simulink model "Simulation_ipmsm_velocity_control"  (R2023a)
settings: Solver=FixedStepDiscrete  StartTime=0.0  StopTime=2  FixedStep=Ts  RelTol=1e-3  EnableMultiTasking=on
PreLoadFcn:
  | ee_ipmsm_velocity_control_data;
StopFcn:
  | ee_addSimlogTimeStamp(bdroot)
undefined symbols (not defined in the file): Ld, Lq, p, psim, Ts, VDC_VECT, Vnom
libraries: nesl_utility x14, fl_lib x11, mcbcontrolslib x9, ee_lib x4, simulink x2, batteryecm_lib x1, eePmsmCurrentController x1, eeTransforms x1, eePmsmCurrentReferenceGen x1, eeVelocityController x1, eePwmGeneratorTwoLevel x1, SignalEditorBlockLib x1
(part 2 of 2)

== system Simulation_ipmsm_velocity_control/Control/Current Control/Subsystem1/Subsystem2/HPF_Calc ==
  In1 : Inport
  VfHpf_FilterCornerFreq_Hz : Inport  Port=2
  VfHpf_FilterTs_s : Inport  Port=3
  HPF_Coef_Calc : Subsystem
  HPF_Module : Subsystem
  HPF : Outport
  wires:
  VfHpf_FilterCornerFreq_Hz/1 -> HPF_Coef_Calc/1(VfHpf_FilterCornerFreq_Hz)
  HPF_Coef_Calc/2(VfHpf_FilterD_coef) -> HPF_Module/3(VfHpf_FilterD_coef)
  HPF_Coef_Calc/1(VfHpf_FilterN_coef) -> HPF_Module/2(VfHpf_FilterN_coef)
  HPF_Module/1(HPF) -> HPF/1
  In1/1 -> HPF_Module/1(In1)
  VfHpf_FilterTs_s/1 -> HPF_Coef_Calc/2(VfHpf_FilterTs_s)

== system Simulation_ipmsm_velocity_control/Control/Current Control/Subsystem1/Subsystem3/HPF_Calc ==
  In1 : Inport
  VfHpf_FilterCornerFreq_Hz : Inport  Port=2
  VfHpf_FilterTs_s : Inport  Port=3
  HPF_Coef_Calc : Subsystem
  HPF_Module : Subsystem
  HPF : Outport
  wires:
  VfHpf_FilterCornerFreq_Hz/1 -> HPF_Coef_Calc/1(VfHpf_FilterCornerFreq_Hz)
  HPF_Coef_Calc/2(VfHpf_FilterD_coef) -> HPF_Module/3(VfHpf_FilterD_coef)
  HPF_Coef_Calc/1(VfHpf_FilterN_coef) -> HPF_Module/2(VfHpf_FilterN_coef)
  HPF_Module/1(HPF) -> HPF/1
  In1/1 -> HPF_Module/1(In1)
  VfHpf_FilterTs_s/1 -> HPF_Coef_Calc/2(VfHpf_FilterTs_s)

== system Simulation_ipmsm_velocity_control/Control/Current Control/SVM_PU/T1_T2_Calc/Subsystem1/Enabled Subsystem ==
  Z : Inport
  Y : Inport  Port=2
  Action Port : ActionPort  ActionPortLabel=case [ 1 ]:
  T4 : Outport
  T6 : Outport  Port=2
  wires:
  Z/1 -> T4/1
  Y/1 -> T6/1

== system Simulation_ipmsm_velocity_control/Control/Current Control/SVM_PU/T1_T2_Calc/Subsystem1/Enabled Subsystem1 ==
  Y : Inport
  X : Inport  Port=2
  Action Port : ActionPort  ActionPortLabel=case [ 2 ]:
  Gain : Gain  Gain=-1
  T4 : Outport
  T6 : Outport  Port=2
  wires:
  Y/1 -> T4/1
  Gain/1 -> T6/1
  X/1 -> Gain/1

== system Simulation_ipmsm_velocity_control/Control/Current Control/SVM_PU/T1_T2_Calc/Subsystem1/Enabled Subsystem2 ==
  Z : Inport
  X : Inport  Port=2
  Action Port : ActionPort  ActionPortLabel=case [ 3 ]:
  Gain : Gain  Gain=-1
  T4 : Outport
  T6 : Outport  Port=2
  wires:
  Z/1 -> Gain/1
  X/1 -> T6/1
  Gain/1 -> T4/1

== system Simulation_ipmsm_velocity_control/Control/Current Control/SVM_PU/T1_T2_Calc/Subsystem1/Enabled Subsystem3 ==
  X : Inport
  Z : Inport  Port=2
  Action Port : ActionPort  ActionPortLabel=case [ 4 ]:
  Gain : Gain  Gain=-1
  T4 : Outport
  T6 : Outport  Port=2
  wires:
  X/1 -> Gain/1
  Z/1 -> T6/1
  Gain/1 -> T4/1

== system Simulation_ipmsm_velocity_control/Control/Current Control/SVM_PU/T1_T2_Calc/Subsystem1/Enabled Subsystem4 ==
  X : Inport
  Y : Inport  Port=2
  Action Port : ActionPort  ActionPortLabel=case [ 5 ]:
  Gain : Gain  Gain=-1
  T4 : Outport
  T6 : Outport  Port=2
  wires:
  Y/1 -> Gain/1
  X/1 -> T4/1
  Gain/1 -> T6/1

== system Simulation_ipmsm_velocity_control/Control/Current Control/SVM_PU/T1_T2_Calc/Subsystem1/Enabled Subsystem5 ==
  Y : Inport
  Z : Inport  Port=2
  Action Port : ActionPort  ActionPortLabel=case [ 6 ]:
  Gain : Gain  Gain=-1
  Gain1 : Gain  Gain=-1
  T4 : Outport
  T6 : Outport  Port=2
  wires:
  Y/1 -> Gain/1
  Z/1 -> Gain1/1
  Gain/1 -> T4/1
  Gain1/1 -> T6/1

== system Simulation_ipmsm_velocity_control/Control/Current Control/SVM_PU/T1_T2_Calc/Subsystem1/Enabled Subsystem6 ==
  Y : Inport
  Z : Inport  Port=2
  Action Port : ActionPort  ActionPortLabel=default:
  Gain : Gain  Gain=-1
  Gain1 : Gain  Gain=-1
  T4 : Outport
  T6 : Outport  Port=2
  wires:
  Y/1 -> Gain/1
  Z/1 -> Gain1/1
  Gain/1 -> T4/1
  Gain1/1 -> T6/1

== system Simulation_ipmsm_velocity_control/Control/Current Control/SVM_PU/T1_T2_Calc/Subsystem2/If Action Subsystem ==
  Bus_T4T6 : Inport
  Action Port : ActionPort  ActionPortLabel=else
  Bus Selector : BusSelector  OutputSignals=T4,T6
  Signal Copy1 : SignalConversion  OverrideOpt=off
  Signal Copy2 : SignalConversion  OverrideOpt=off
  T1 : Outport
  T2 : Outport  Port=2
  wires:
  Bus_T4T6/1 -> Bus Selector/1
  Bus Selector/1 -> Signal Copy1/1  "<T4>"
  Bus Selector/2 -> Signal Copy2/1  "<T6>"
  Signal Copy1/1 -> T1/1
  Signal Copy2/1 -> T2/1

== system Simulation_ipmsm_velocity_control/Control/Current Control/SVM_PU/T1_T2_Calc/Subsystem2/If Action Subsystem1 ==
  Bus_T4T6 : Inport
  Action Port : ActionPort  ActionPortLabel=elseif(u1 > 1)
  Add : Sum
  Bus Selector : BusSelector  OutputSignals=T4,T6
  Divide : Product  Inputs=*/
  Divide1 : Product  Inputs=/*
  T1 : Outport
  T2 : Outport  Port=2
  wires:
  Bus_T4T6/1 -> Bus Selector/1
  Bus Selector/1 -> Divide/1, Add/1  "<T4>"
  Bus Selector/2 -> Divide1/2, Add/2  "<T6>"
  Add/1 -> Divide1/1, Divide/2
  Divide/1 -> T1/1  "T1"
  Divide1/1 -> T2/1  "T2"

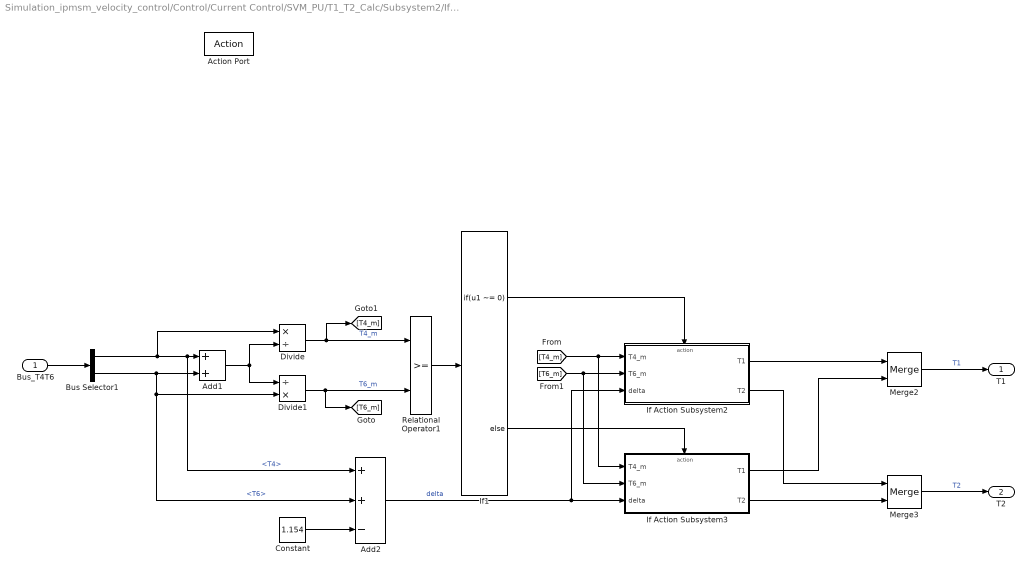
== system Simulation_ipmsm_velocity_control/Control/Current Control/SVM_PU/T1_T2_Calc/Subsystem2/If Action Subsystem2 ==
  Bus_T4T6 : Inport
  Action Port : ActionPort  ActionPortLabel=if(u1 > 1.154 )
  Add1 : Sum
  Add2 : Sum  Inputs=++-
  Bus Selector1 : BusSelector  OutputSignals=T4,T6
  Constant : Constant  Value=1.154  OutDataTypeStr=single
  Divide : Product  Inputs=*/
  Divide1 : Product  Inputs=/*
  If Action Subsystem2 : Subsystem  TreatAsAtomicUnit=on
  If Action Subsystem3 : Subsystem  TreatAsAtomicUnit=on
  If1 : If  IfExpression=u1 ~= 0
  Merge2 : Merge
  Merge3 : Merge
  Relational Operator1 : RelationalOperator  OutDataTypeStr=boolean  RndMeth=Simplest  InputSameDT=off
  T1 : Outport
  T2 : Outport  Port=2
  wires:
  Bus_T4T6/1 -> Bus Selector1/1
  Bus Selector1/2 -> Divide1/2, Add2/2, Add1/2  "<T6>"
  Divide/1 -> [T4_m], Relational Operator1/1  "T4_m"
  Bus Selector1/1 -> Divide/1, Add2/1, Add1/1  "<T4>"
  Divide1/1 -> [T6_m], Relational Operator1/2  "T6_m"
  Add1/1 -> Divide1/1, Divide/2
  Relational Operator1/1 -> If1/1
  Constant/1 -> Add2/3
  Add2/1 -> If Action Subsystem2/3(delta), If Action Subsystem3/3(delta)  "delta"
  If1/1 -> If Action Subsystem2/Action
  If1/2 -> If Action Subsystem3/Action
  If Action Subsystem2/1(T1) -> Merge2/1
  If Action Subsystem3/1(T1) -> Merge2/2
  If Action Subsystem3/2(T2) -> Merge3/2
  If Action Subsystem2/2(T2) -> Merge3/1
  Merge2/1 -> T1/1  "T1"
  Merge3/1 -> T2/1  "T2"
  [T4_m] -> If Action Subsystem3/1(T4_m), If Action Subsystem2/1(T4_m)
  [T6_m] -> If Action Subsystem3/2(T6_m), If Action Subsystem2/2(T6_m)

== system Simulation_ipmsm_velocity_control/Control/Current Control/Subsystem1/Subsystem2/HPF_Calc/HPF_Coef_Calc ==
  VfHpf_FilterCornerFreq_Hz : Inport
  VfHpf_FilterTs_s : Inport  Port=2
  Add : Sum
  Add1 : Sum  Inputs=+-
  Constant : Constant  Value=2*pi  OutDataTypeStr=single
  Constant1 : Constant  Value=2  OutDataTypeStr=single
  Divide : Product  Inputs=*/
  Divide1 : Product  Inputs=/*
  Product : Product  Inputs=3
  VfHpf_FilterN_coef : Outport
  VfHpf_FilterD_coef : Outport  Port=2
  wires:
  VfHpf_FilterCornerFreq_Hz/1 -> Product/1
  VfHpf_FilterTs_s/1 -> Product/2
  Constant/1 -> Product/3
  Product/1 -> Add1/2, Add/2  "Omiga0PrTs"
  Constant1/1 -> Add1/1, Divide/1, Add/1
  Add/1 -> Divide1/1, Divide/2
  Divide/1 -> VfHpf_FilterN_coef/1
  Add1/1 -> Divide1/2
  Divide1/1 -> VfHpf_FilterD_coef/1

== system Simulation_ipmsm_velocity_control/Control/Current Control/Subsystem1/Subsystem2/HPF_Calc/HPF_Module ==
  In1 : Inport
  VfHpf_FilterN_coef : Inport  Port=2
  VfHpf_FilterD_coef : Inport  Port=3
  Add : Sum  Inputs=+-
  Add1 : Sum
  Delay : Delay  DelayLength=1
  Delay1 : Delay  DelayLength=1
  Product : Product
  Product1 : Product
  HPF : Outport
  wires:
  In1/1 -> Delay/1, Add/1
  Delay/1 -> Add/2
  Add/1 -> Product/1
  VfHpf_FilterN_coef/1 -> Product/2
  Product/1 -> Add1/1
  Add1/1 -> Delay1/1, HPF/1
  VfHpf_FilterD_coef/1 -> Product1/1
  Product1/1 -> Add1/2
  Delay1/1 -> Product1/2

== system Simulation_ipmsm_velocity_control/Control/Current Control/Subsystem1/Subsystem3/HPF_Calc/HPF_Coef_Calc ==
  VfHpf_FilterCornerFreq_Hz : Inport
  VfHpf_FilterTs_s : Inport  Port=2
  Add : Sum
  Add1 : Sum  Inputs=+-
  Constant : Constant  Value=2*pi  OutDataTypeStr=single
  Constant1 : Constant  Value=2  OutDataTypeStr=single
  Divide : Product  Inputs=*/
  Divide1 : Product  Inputs=/*
  Product : Product  Inputs=3
  VfHpf_FilterN_coef : Outport
  VfHpf_FilterD_coef : Outport  Port=2
  wires:
  VfHpf_FilterCornerFreq_Hz/1 -> Product/1
  VfHpf_FilterTs_s/1 -> Product/2
  Constant/1 -> Product/3
  Product/1 -> Add1/2, Add/2  "Omiga0PrTs"
  Constant1/1 -> Add1/1, Divide/1, Add/1
  Add/1 -> Divide1/1, Divide/2
  Divide/1 -> VfHpf_FilterN_coef/1
  Add1/1 -> Divide1/2
  Divide1/1 -> VfHpf_FilterD_coef/1

== system Simulation_ipmsm_velocity_control/Control/Current Control/Subsystem1/Subsystem3/HPF_Calc/HPF_Module ==
  In1 : Inport
  VfHpf_FilterN_coef : Inport  Port=2
  VfHpf_FilterD_coef : Inport  Port=3
  Add : Sum  Inputs=+-
  Add1 : Sum
  Delay : Delay  DelayLength=1
  Delay1 : Delay  DelayLength=1
  Product : Product
  Product1 : Product
  HPF : Outport
  wires:
  In1/1 -> Delay/1, Add/1
  Delay/1 -> Add/2
  Add/1 -> Product/1
  VfHpf_FilterN_coef/1 -> Product/2
  Product/1 -> Add1/1
  Add1/1 -> Delay1/1, HPF/1
  VfHpf_FilterD_coef/1 -> Product1/1
  Product1/1 -> Add1/2
  Delay1/1 -> Product1/2

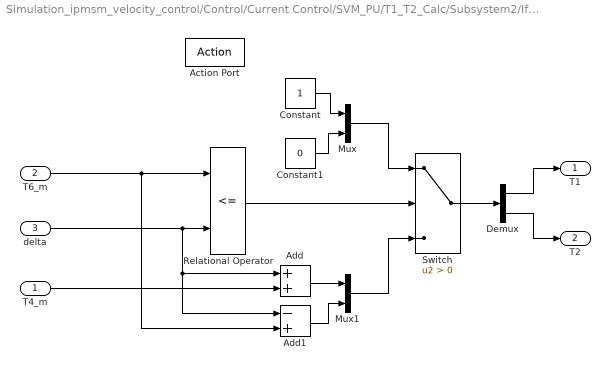
== system Simulation_ipmsm_velocity_control/Control/Current Control/SVM_PU/T1_T2_Calc/Subsystem2/If Action Subsystem2/If Action Subsystem2 ==
  T4_m : Inport
  T6_m : Inport  Port=2
  delta : Inport  Port=3
  Action Port : ActionPort  ActionPortLabel=if(u1 ~= 0)
  Add : Sum
  Add1 : Sum  Inputs=-+
  Constant : Constant  OutDataTypeStr=single
  Constant1 : Constant  Value=0  OutDataTypeStr=single
  Demux : Demux  Outputs=2
  Mux : Mux  Inputs=2
  Mux1 : Mux  Inputs=2
  Relational Operator : RelationalOperator  Operator=<=  OutDataTypeStr=boolean  RndMeth=Simplest  InputSameDT=off
  Switch : Switch  Criteria=u2 > Threshold  SaturateOnIntegerOverflow=off  InputSameDT=off
  T1 : Outport
  T2 : Outport  Port=2
  wires:
  T6_m/1 -> Add1/2, Relational Operator/1
  delta/1 -> Add/1, Add1/1, Relational Operator/2
  Relational Operator/1 -> Switch/2
  Constant/1 -> Mux/1
  Constant1/1 -> Mux/2
  Mux/1 -> Switch/1
  T4_m/1 -> Add/2
  Add/1 -> Mux1/1
  Add1/1 -> Mux1/2
  Mux1/1 -> Switch/3
  Switch/1 -> Demux/1
  Demux/1 -> T1/1
  Demux/2 -> T2/1

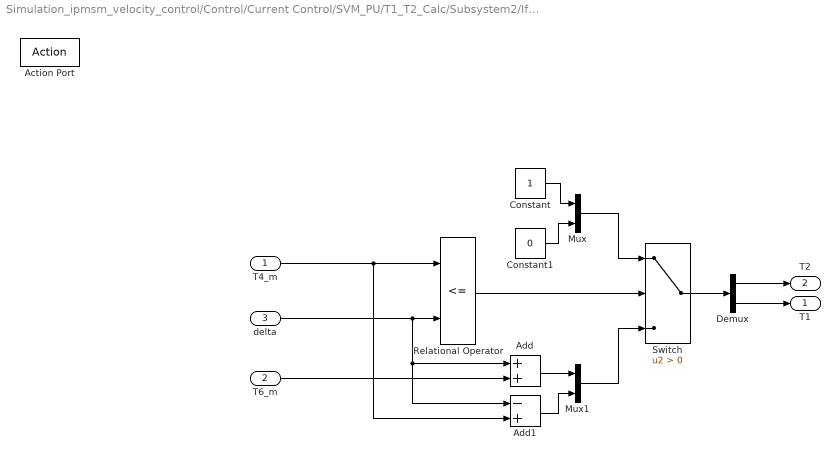
== system Simulation_ipmsm_velocity_control/Control/Current Control/SVM_PU/T1_T2_Calc/Subsystem2/If Action Subsystem2/If Action Subsystem3 ==
  T4_m : Inport
  T6_m : Inport  Port=2
  delta : Inport  Port=3
  Action Port : ActionPort  ActionPortLabel=else
  Add : Sum
  Add1 : Sum  Inputs=-+
  Constant : Constant  OutDataTypeStr=single
  Constant1 : Constant  Value=0  OutDataTypeStr=single
  Demux : Demux  Outputs=2
  Mux : Mux  Inputs=2
  Mux1 : Mux  Inputs=2
  Relational Operator : RelationalOperator  Operator=<=  OutDataTypeStr=boolean  RndMeth=Simplest  InputSameDT=off
  Switch : Switch  Criteria=u2 > Threshold  SaturateOnIntegerOverflow=off  InputSameDT=off
  T1 : Outport
  T2 : Outport  Port=2
  wires:
  Mux1/1 -> Switch/3
  delta/1 -> Add/1, Add1/1, Relational Operator/2
  Add1/1 -> Mux1/2
  Mux/1 -> Switch/1
  Relational Operator/1 -> Switch/2
  Switch/1 -> Demux/1
  Constant1/1 -> Mux/2
  Add/1 -> Mux1/1
  Constant/1 -> Mux/1
  T4_m/1 -> Add1/2, Relational Operator/1
  T6_m/1 -> Add/2
  Demux/2 -> T1/1
  Demux/1 -> T2/1

== stateflow chart Simulation_ipmsm_velocity_control/Control/Task Scheduler ==
  (default) -> (junction 23) : CLK_50us
  (junction 23) -> (junction 17)
  (junction 17) -> (junction 22) [order 2]
  (junction 17) -> (junction 22) [order 1] : [cnt%%2==0]{Task_100us_1;}
  (junction 22) -> (junction 18) [order 2]
  (junction 22) -> (junction 18) [order 1] : [cnt%%2==0]{Task_100us_2;}
  (junction 18) -> (junction 21) [order 1] : [cnt%%20==0]{Task_1ms_1;}
  (junction 18) -> (junction 21) [order 2]
  (junction 21) -> (junction 34) [order 2]
  (junction 21) -> (junction 16) [order 1] : [1]{cnt++;}
  data: cnt local int32
  events: Task_100us_1 output FUNCTION_CALL_EVENT; Task_100us_2 output FUNCTION_CALL_EVENT; Task_1ms_1 output FUNCTION_CALL_EVENT; CLK_50us input FUNCTION_CALL_EVENT
